simulink model "posModel3"  (R2021b)
settings: Solver=ode5  StartTime=0.0  StopTime=131.071  FixedStep=dt  RelTol=1e-3
values from neighbouring files (symbols this model uses):
  A = [0 1; 0 -Bm/Jm]    [posInit3.m]
  B = [0; 1/Jm]    [posInit3.m]
  Bm = bm * gearRatio * gearRatio    (= 2.601)    [posInit1.m]    (also in posInit2.m; posInit3.m)
  C = [1, 0]    [posInit3.m]
  dcGain = - C * inv(A - B * [kp, 0]) * B    [posInit3.m]
  Jm = jm * gearRatio * gearRatio    (= 0.023968215)    [posInit1.m]    (also in posInit2.m; posInit3.m)
  kp = 50    [posInit1.m]    (also in posInit2.m; posInit3.m = 80)
  ssConCloseLoop = ss(A - B * [kp, 0],B,C,D)    [posInit3.m]
  ssDisCloseLoop = c2d(ssConCloseLoop,0.001)    [posInit3.m]
libraries: simulink x1
settings Model: Creator=86135  LastModifiedBy=86135

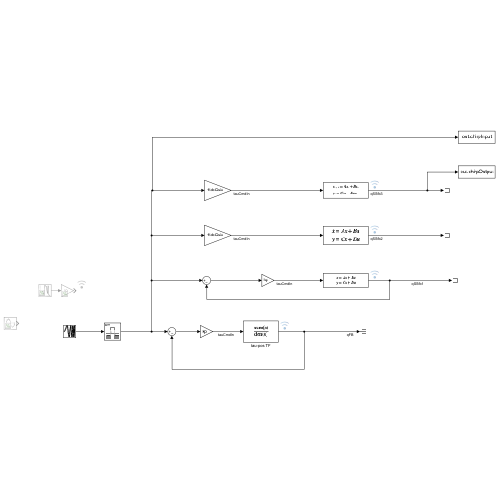
[thumbnail: Simulink's stored preview of the top-level diagram]
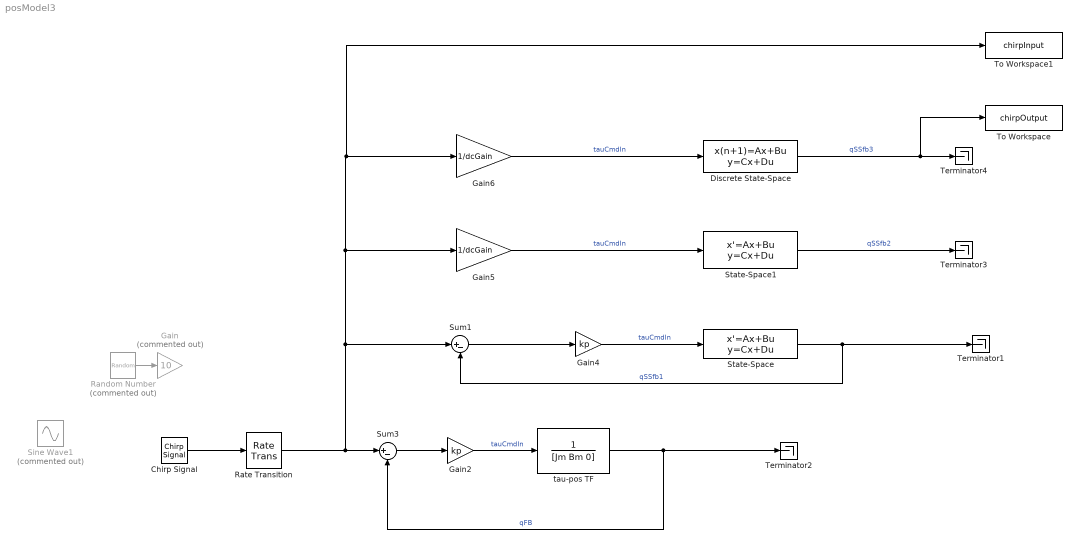
== system posModel3 ==
  Chirp Signal : simulink/Sources/Chirp Signal  f1=f0  T=131.071  f2=f1
  Discrete State-Space : DiscreteStateSpace  A=ssDisCloseLoop.A  B=ssDisCloseLoop.B  C=ssDisCloseLoop.C  D=ssDisCloseLoop.D  SampleTime=0.001
  Gain : Gain  Commented=on  Gain=10
  Gain2 : Gain  Gain=kp
  Gain4 : Gain  Gain=kp
  Gain5 : Gain  Gain=1/dcGain
  Gain6 : Gain  Gain=1/dcGain
  Random Number : RandomNumber  Commented=on  Variance=10  Seed=11111  SampleTime=0.5
  Rate Transition : RateTransition  Deterministic=off  OutPortSampleTime=0.001
  Sine Wave1 : Sin  Commented=on  Frequency=23  SampleTime=0
  State-Space : StateSpace  A=A  B=B  C=C  D=0  InitialCondition=0
  State-Space1 : StateSpace  A=ssConCloseLoop.A  B=ssConCloseLoop.B  C=ssConCloseLoop.C  D=ssConCloseLoop.D  InitialCondition=0  ParameterTunability=Optimized
  Sum1 : Sum  Inputs=|+-
  Sum3 : Sum  Inputs=|+-
  Terminator{1..4} (4 alike) : Terminator
  To Workspace : ToWorkspace  VariableName=chirpOutput  SaveFormat=Timeseries  SampleTime=-1
  To Workspace1 : ToWorkspace  VariableName=chirpInput  SaveFormat=Timeseries  SampleTime=-1
  tau-pos TF : TransferFcn  Denominator=[Jm Bm 0]
  wires:
  Sum3/1 -> Gain2/1
  Gain2/1 -> tau-pos TF/1  "tauCmdIn"
  tau-pos TF/1 -> Terminator2/1, Sum3/2  "qFB"
  Gain4/1 -> State-Space/1  "tauCmdIn"
  Sum1/1 -> Gain4/1
  State-Space/1 -> Terminator1/1, Sum1/2  "qSSfb1"
  State-Space1/1 -> Terminator3/1  "qSSfb2"
  Discrete State-Space/1 -> To Workspace/1, Terminator4/1  "qSSfb3"
  Rate Transition/1 -> Sum3/1, To Workspace1/1, Gain6/1, Gain5/1, Sum1/1
  Gain5/1 -> State-Space1/1  "tauCmdIn"
  Gain6/1 -> Discrete State-Space/1  "tauCmdIn"
  Random Number/1 -> Gain/1
  Chirp Signal/1 -> Rate Transition/1
